simulink model "HLSDem_SetPoint"  (R2016b)
settings: configuration reference "CodeGenConfigSet" (kept outside this file)
values from neighbouring files (symbols this model uses):
  EPM_N_MAX = fi(10000,EngSpeed_rpm)    [init_HLSDem_SetPoint.m]    (also in init_HLSDem_SetPoint_SIL.m)
  HLSDem_dnSetPLoLimHiTrm_C = Calibration.Parameter    [init_HLSDem_SetPoint.m]    (also in init_HLSDem_SetPoint_SIL.m = Simulink.Parameter)
  HLSDem_dnSetPLoLimLoTrm_C = Calibration.Parameter    [init_HLSDem_SetPoint.m]    (also in init_HLSDem_SetPoint_SIL.m = Simulink.Parameter)
  HLSDem_facFdbkCANKick_C = Calibration.Parameter    [init_HLSDem_SetPoint.m]    (also in init_HLSDem_SetPoint_SIL.m = Simulink.Parameter)
  HLSDem_facFdbkDrvKick_C = Calibration.Parameter    [init_HLSDem_SetPoint.m]    (also in init_HLSDem_SetPoint_SIL.m = Simulink.Parameter)
  HLSDem_facFdbkHGG_C = Calibration.Parameter    [init_HLSDem_SetPoint.m]    (also in init_HLSDem_SetPoint_SIL.m = Simulink.Parameter)
  HLSDem_facFdbkLGG_C = Calibration.Parameter    [init_HLSDem_SetPoint.m]    (also in init_HLSDem_SetPoint_SIL.m = Simulink.Parameter)
  HLSDem_facFdbkMaxAcs_C = Calibration.Parameter    [init_HLSDem_SetPoint.m]    (also in init_HLSDem_SetPoint_SIL.m = Simulink.Parameter)
  HLSDem_facFdbkMaxSysErr_C = Calibration.Parameter    [init_HLSDem_SetPoint.m]    (also in init_HLSDem_SetPoint_SIL.m = Simulink.Parameter)
  HLSDem_facFdbkMaxTra_C = Calibration.Parameter    [init_HLSDem_SetPoint.m]    (also in init_HLSDem_SetPoint_SIL.m = Simulink.Parameter)
  HLSDem_facFdbkRed1_C = Calibration.Parameter    [init_HLSDem_SetPoint.m]    (also in init_HLSDem_SetPoint_SIL.m = Simulink.Parameter)
  HLSDem_facFdbkRed2_C = Calibration.Parameter    [init_HLSDem_SetPoint.m]    (also in init_HLSDem_SetPoint_SIL.m = Simulink.Parameter)
  HLSDem_facFdbkRed3_C = Calibration.Parameter    [init_HLSDem_SetPoint.m]    (also in init_HLSDem_SetPoint_SIL.m = Simulink.Parameter)
  HLSDem_facFdbkStrt_C = Calibration.Parameter    [init_HLSDem_SetPoint.m]    (also in init_HLSDem_SetPoint_SIL.m = Simulink.Parameter)
  HLSDem_facFdbkSysDgrt1_C = Calibration.Parameter    [init_HLSDem_SetPoint.m]    (also in init_HLSDem_SetPoint_SIL.m = Simulink.Parameter)
  HLSDem_facFdbkSysDgrt2_C = Calibration.Parameter    [init_HLSDem_SetPoint.m]    (also in init_HLSDem_SetPoint_SIL.m = Simulink.Parameter)
  HLSDem_facFdbkSysDgrt3_C = Calibration.Parameter    [init_HLSDem_SetPoint.m]    (also in init_HLSDem_SetPoint_SIL.m = Simulink.Parameter)
  HLSDem_facSetPLoFlt_C = Calibration.Parameter    [init_HLSDem_SetPoint.m]    (also in init_HLSDem_SetPoint_SIL.m = Simulink.Parameter)
  HLSDem_facTrqHiPT1_C = Calibration.Parameter    [init_HLSDem_SetPoint.m]    (also in init_HLSDem_SetPoint_SIL.m = Simulink.Parameter)
  HLSDem_facTrqLoPT1_C = Calibration.Parameter    [init_HLSDem_SetPoint.m]    (also in init_HLSDem_SetPoint_SIL.m = Simulink.Parameter)
  HLSDem_nHGGSetPHi_C = Calibration.Parameter    [init_HLSDem_SetPoint.m]    (also in init_HLSDem_SetPoint_SIL.m = Simulink.Parameter)
  HLSDem_nKDSetPHi_C = Calibration.Parameter    [init_HLSDem_SetPoint.m]    (also in init_HLSDem_SetPoint_SIL.m = Simulink.Parameter)
  HLSDem_nLGGSetPHi_C = Calibration.Parameter    [init_HLSDem_SetPoint.m]    (also in init_HLSDem_SetPoint_SIL.m = Simulink.Parameter)
  HLSDem_nRed1SetPHi_C = Calibration.Parameter    [init_HLSDem_SetPoint.m]    (also in init_HLSDem_SetPoint_SIL.m = Simulink.Parameter)
  HLSDem_nRed2SetPHi_C = Calibration.Parameter    [init_HLSDem_SetPoint.m]    (also in init_HLSDem_SetPoint_SIL.m = Simulink.Parameter)
  HLSDem_nRed3SetPHi_C = Calibration.Parameter    [init_HLSDem_SetPoint.m]    (also in init_HLSDem_SetPoint_SIL.m = Simulink.Parameter)
  HLSDem_nSel1SetPLo_C = Calibration.Parameter    [init_HLSDem_SetPoint.m]    (also in init_HLSDem_SetPoint_SIL.m = Simulink.Parameter)
  HLSDem_nSel2SetPLo_C = Calibration.Parameter    [init_HLSDem_SetPoint.m]    (also in init_HLSDem_SetPoint_SIL.m = Simulink.Parameter)
  HLSDem_nSel3SetPLo_C = Calibration.Parameter    [init_HLSDem_SetPoint.m]    (also in init_HLSDem_SetPoint_SIL.m = Simulink.Parameter)
  HLSDem_nSetPLoDia_C = Calibration.Parameter    [init_HLSDem_SetPoint.m]    (also in init_HLSDem_SetPoint_SIL.m = Simulink.Parameter)
  HLSDem_nSetPLoDrvAwy_C = Calibration.Parameter    [init_HLSDem_SetPoint.m]    (also in init_HLSDem_SetPoint_SIL.m = Simulink.Parameter)
  HLSDem_nSetPLoIni_CUR = Calibration.Parameter    [init_HLSDem_SetPoint.m]    (also in init_HLSDem_SetPoint_SIL.m = Simulink.Parameter)
  HLSDem_nSetPLoIni_CURX = Calibration.Parameter    [init_HLSDem_SetPoint.m]    (also in init_HLSDem_SetPoint_SIL.m = Simulink.Parameter)
  HLSDem_nSetPLoMax_C = Calibration.Parameter    [init_HLSDem_SetPoint.m]    (also in init_HLSDem_SetPoint_SIL.m = Simulink.Parameter)
  HLSDem_nSetPLoMaxOfs_C = Calibration.Parameter    [init_HLSDem_SetPoint.m]    (also in init_HLSDem_SetPoint_SIL.m = Simulink.Parameter)
  HLSDem_nSetPLoOfsMoF_C = Calibration.Parameter    [init_HLSDem_SetPoint.m]    (also in init_HLSDem_SetPoint_SIL.m = Simulink.Parameter)
  HLSDem_nSetPLoWrm_C = Calibration.Parameter    [init_HLSDem_SetPoint.m]    (also in init_HLSDem_SetPoint_SIL.m = Simulink.Parameter)
  HLSDem_nSpdLowBattUAdd_CUR = Calibration.Parameter    [init_HLSDem_SetPoint.m]    (also in init_HLSDem_SetPoint_SIL.m = Simulink.Parameter)
  HLSDem_nSpdLowBattUAdd_CURX = Calibration.Parameter    [init_HLSDem_SetPoint.m]    (also in init_HLSDem_SetPoint_SIL.m = Simulink.Parameter)
  HLSDem_nSpdLowBattUAddLim_C = Calibration.Parameter    [init_HLSDem_SetPoint.m]    (also in init_HLSDem_SetPoint_SIL.m = Simulink.Parameter)
  HLSDem_nStrtSetPHi_C = Calibration.Parameter    [init_HLSDem_SetPoint.m]    (also in init_HLSDem_SetPoint_SIL.m = Simulink.Parameter)
  HLSDem_nSysDgrtSetPHi_C = Calibration.Parameter    [init_HLSDem_SetPoint.m]    (also in init_HLSDem_SetPoint_SIL.m = Simulink.Parameter)
  HLSDem_rTrqSwt_C = Calibration.Parameter    [init_HLSDem_SetPoint.m]    (also in init_HLSDem_SetPoint_SIL.m = Simulink.Parameter)
  HLSDem_SetPHiRmpSlopeNeg_C = Calibration.Parameter    [init_HLSDem_SetPoint.m]    (also in init_HLSDem_SetPoint_SIL.m = Simulink.Parameter)
  HLSDem_SetPHiRmpSlopePos_C = Calibration.Parameter    [init_HLSDem_SetPoint.m]    (also in init_HLSDem_SetPoint_SIL.m = Simulink.Parameter)
  HLSDem_SetPLoRmpSlopeNeg_C = Calibration.Parameter    [init_HLSDem_SetPoint.m]    (also in init_HLSDem_SetPoint_SIL.m = Simulink.Parameter)
  HLSDem_SetPLoRmpSlopePos_C = Calibration.Parameter    [init_HLSDem_SetPoint.m]    (also in init_HLSDem_SetPoint_SIL.m = Simulink.Parameter)
  HLSDem_SetPLoTipInRmpSlopeNeg_C = Calibration.Parameter    [init_HLSDem_SetPoint.m]    (also in init_HLSDem_SetPoint_SIL.m = Simulink.Parameter)
  HLSDem_SetPLoTipInRmpSlopePos_C = Calibration.Parameter    [init_HLSDem_SetPoint.m]    (also in init_HLSDem_SetPoint_SIL.m = Simulink.Parameter)
  HLSDem_stSetPLoFlt_C = Calibration.Parameter    [init_HLSDem_SetPoint.m]    (also in init_HLSDem_SetPoint_SIL.m = Simulink.Parameter)
  HLSDem_stSpdSel_C = Calibration.Parameter    [init_HLSDem_SetPoint.m]    (also in init_HLSDem_SetPoint_SIL.m = Simulink.Parameter)
  HLSDem_stSysDgrtSetPHi_C = Calibration.Parameter    [init_HLSDem_SetPoint.m]    (also in init_HLSDem_SetPoint_SIL.m = Simulink.Parameter)
  HLSDem_swtDisblVehIfcSetPHi_C = Calibration.Parameter    [init_HLSDem_SetPoint.m]    (also in init_HLSDem_SetPoint_SIL.m = Simulink.Parameter)
  HLSDem_swtEnaPTO_C = Calibration.Parameter    [init_HLSDem_SetPoint.m]    (also in init_HLSDem_SetPoint_SIL.m = Simulink.Parameter)
  HLSDem_swtMode_C = Calibration.Parameter    [init_HLSDem_SetPoint.m]    (also in init_HLSDem_SetPoint_SIL.m = Simulink.Parameter)
  HLSDem_swtTempSel_C = Calibration.Parameter    [init_HLSDem_SetPoint.m]    (also in init_HLSDem_SetPoint_SIL.m = Simulink.Parameter)
  HLSDem_swtTrqHiSel_C = Calibration.Parameter    [init_HLSDem_SetPoint.m]    (also in init_HLSDem_SetPoint_SIL.m = Simulink.Parameter)
  HLSDem_swtTrqLoSel_C = Calibration.Parameter    [init_HLSDem_SetPoint.m]    (also in init_HLSDem_SetPoint_SIL.m = Simulink.Parameter)
  HLSDem_tDflSetPLo_C = Calibration.Parameter    [init_HLSDem_SetPoint.m]    (also in init_HLSDem_SetPoint_SIL.m = Simulink.Parameter)
  HLSDem_tiMaxIncrSetPLo_C = Calibration.Parameter    [init_HLSDem_SetPoint.m]    (also in init_HLSDem_SetPoint_SIL.m = Simulink.Parameter)
  HLSDem_tiSpdLowBattUAdd_C = Calibration.Parameter    [init_HLSDem_SetPoint.m]    (also in init_HLSDem_SetPoint_SIL.m = Simulink.Parameter)
  HLSDem_tiStrtCEngDsT_CUR = Calibration.Parameter    [init_HLSDem_SetPoint.m]    (also in init_HLSDem_SetPoint_SIL.m = Simulink.Parameter)
  HLSDem_tiStrtCEngDsT_CURX = Calibration.Parameter    [init_HLSDem_SetPoint.m]    (also in init_HLSDem_SetPoint_SIL.m = Simulink.Parameter)
  HLSDem_tiStrtEngOil_CUR = Calibration.Parameter    [init_HLSDem_SetPoint.m]    (also in init_HLSDem_SetPoint_SIL.m = Simulink.Parameter)
  HLSDem_tiStrtEngOil_CURX = Calibration.Parameter    [init_HLSDem_SetPoint.m]    (also in init_HLSDem_SetPoint_SIL.m = Simulink.Parameter)
  HLSDem_tThresDisbl_C = Calibration.Parameter    [init_HLSDem_SetPoint.m]    (also in init_HLSDem_SetPoint_SIL.m = Simulink.Parameter)
  HLSDem_tThresEna_C = Calibration.Parameter    [init_HLSDem_SetPoint.m]    (also in init_HLSDem_SetPoint_SIL.m = Simulink.Parameter)
  HLSDem_volSpdAddHi_C = Calibration.Parameter    [init_HLSDem_SetPoint.m]    (also in init_HLSDem_SetPoint_SIL.m = Simulink.Parameter)
  HLSDem_volSpdAddLo_C = Calibration.Parameter    [init_HLSDem_SetPoint.m]    (also in init_HLSDem_SetPoint_SIL.m = Simulink.Parameter)
  HndBrk_stDebVal_C = Calibration.Parameter    [init_HLSDem_SetPoint.m]    (also in init_HLSDem_SetPoint_SIL.m = Simulink.Parameter)
  SigTst_nSetPHi_C = Calibration.Parameter    [init_HLSDem_SetPoint.m]    (also in init_HLSDem_SetPoint_SIL.m = Simulink.Parameter)
  SigTst_nSetPLo_C = Calibration.Parameter    [init_HLSDem_SetPoint.m]    (also in init_HLSDem_SetPoint_SIL.m = Simulink.Parameter)
  SigTst_swtSetPHi_C = Calibration.Parameter    [init_HLSDem_SetPoint.m]    (also in init_HLSDem_SetPoint_SIL.m = Simulink.Parameter)
  SigTst_swtSetPLo_C = Calibration.Parameter    [init_HLSDem_SetPoint.m]    (also in init_HLSDem_SetPoint_SIL.m = Simulink.Parameter)
undefined symbols (not defined in the file or in its folder): CEngDst_switch_conv, CEngDsT_tTransf_CURX, EngState_conv, HLSDem_SetPoint_DT, StSys_StrtState_conv, Switch_conv
libraries: CXLib x13, simulink x3
(part 1 of 2)
settings Model: SimulationMode=accelerator  Creator=Administrator  LastModifiedBy=xuxingpei
settings ConfigSetRef: SourceLocation=Base Workspace

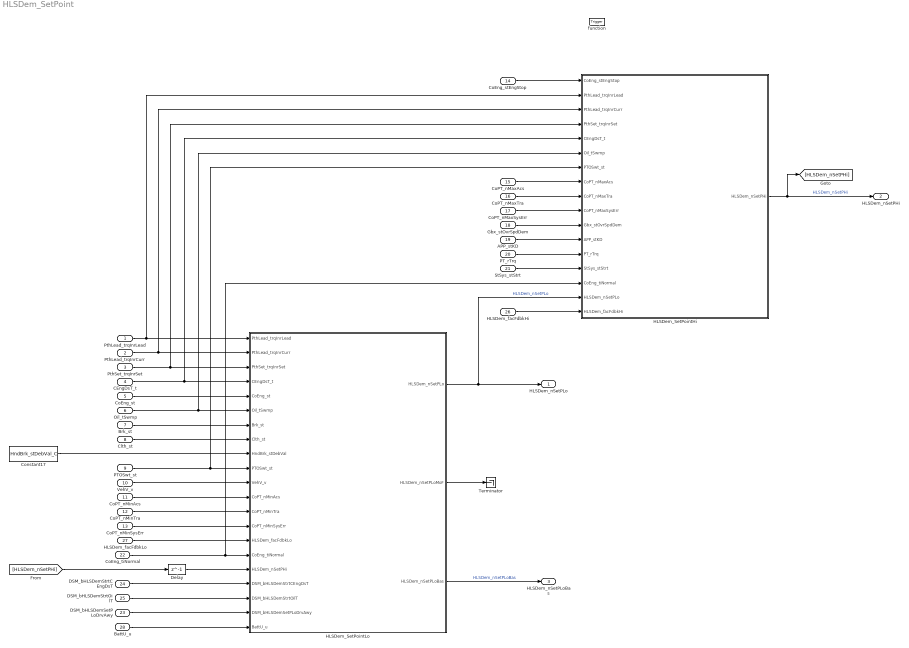
== system HLSDem_SetPoint ==
  PthLead_trqInrLead : Inport  Tag=Nm  Description=Inner torque lead value  OutMin=-3000  OutMax=3000  OutDataTypeStr=Trq_Nm
  PthLead_trqInrCurr : Inport  Tag=Nm  Description=Actual percent engine torque  Port=2  OutMin=-3000  OutMax=3000  OutDataTypeStr=Trq_Nm
  PthSet_trqInrSet : Inport  Tag=Nm  Description=Inner torque set value after monitoring limitation  Port=3  OutMin=-3000  OutMax=3276.7  OutDataTypeStr=Trq_Nm
  CEngDsT_t : Inport  Tag=deg  Description=engine coolant temperature after filter  Port=4  OutMin=-200  OutMax=200  OutDataTypeStr=Temp_deg
  CoEng_st : Inport  Description=Engine coordinator state  Port=5  OutDataTypeStr=Enum: EngState_conv
  Oil_tSwmp : Inport  Tag=deg  Description=Oil temperature in oil sump  Port=6  OutMin=-50  OutMax=200  OutDataTypeStr=Temp_deg
  Brk_st : Inport  Description=Brake switch state  Port=7  OutMin=0  OutMax=255  OutDataTypeStr=State_uint8
  Clth_st : Inport  Description=Clutch information  Port=8  OutMin=0  OutMax=255  OutDataTypeStr=State_uint8
  PTOSwt_st : Inport  Description=Power Take-off switch current state for a specific input voltage  Port=9  OutMin=0  OutMax=255  OutDataTypeStr=State_uint8
  VehV_v : Inport  Tag=km/h  Description=Vehicle speed  Port=10  OutMin=0  OutMax=250  OutDataTypeStr=VehSpeed_km_h
  CoPT_nMinAcs : Inport  Tag=rpm  Description=Application parameter for Minimum engine speed demand of Accessories  Port=11  OutMin=0  OutMax=6000  OutDataTypeStr=EngSpeed_rpm
  CoPT_nMinTra : Inport  Tag=rpm  Description=Application parameter for Minimum engine speed demand of transmission  Port=12  OutMin=0  OutMax=6000  OutDataTypeStr=EngSpeed_rpm
  CoPT_nMinSysErr : Inport  Tag=rpm  Description=Application parameter for Minimum engine speed demand while system error  Port=13  OutMin=0  OutMax=6000  OutDataTypeStr=EngSpeed_rpm
  CoEng_stEngStop : Inport  Description=Bit coded output message from engine stop function for low idle, egine shut off and crank control  Port=14  OutMin=0  OutMax=255  OutDataTypeStr=State_uint8
  CoPT_nMaxAcs : Inport  Tag=rpm  Description=Application parameter for maximum engine speed  Port=15  OutMin=0  OutMax=6000  OutDataTypeStr=EngSpeed_rpm
  CoPT_nMaxTra : Inport  Tag=rpm  Description=Application parameter for maximum engine speed demand of transmission  Port=16  OutMin=0  OutMax=6000  OutDataTypeStr=EngSpeed_rpm
  CoPT_nMaxSysErr : Inport  Tag=rpm  Description=Application parameter for maximum engine speed demand while system error  Port=17  OutMin=0  OutMax=6000  OutDataTypeStr=EngSpeed_rpm
  Gbx_stOvrSpdDem : Inport  Description=status of engine overspeed request  Port=18  OutMin=0  OutMax=255  OutDataTypeStr=State_uint8
  APP_stKD : Inport  Description=State of accelerator pedal kick down  Port=19  OutMin=0  OutMax=1  OutDataTypeStr=boolean
  PT_rTrq : Inport  Description=Powertrain torque ratio  Port=20  OutMin=-100  OutMax=100  OutDataTypeStr=TransRatio
  StSys_stStrt : Inport  Description=state of starting system  Port=21  OutDataTypeStr=Enum: StSys_StrtState_conv
  CoEng_tiNormal : Inport  Tag=ms  Description="Time since state\"CONENG_RUNNING\"was reached"  Port=22  OutMin=0  OutMax=42949672950  OutDataTypeStr=EngTime_ms
  DSM_bHLSDemSetPLoDrvAwy : Inport  Description=Status of FId_HLSDemSetPLoDrvAwy  Port=23  OutMin=0  OutMax=1  OutDataTypeStr=boolean
  DSM_bHLSDemStrtCEngDsT : Inport  Description=Status of FId_HLSDemStrtCEngDsT  Port=24  OutMin=0  OutMax=1  OutDataTypeStr=boolean
  DSM_bHLSDemStrtOilT : Inport  Description=Status of FId_HLSDemStrtOilT  Port=25  OutMin=0  OutMax=1  OutDataTypeStr=boolean
  HLSDem_facFdbkHi : Inport  Tag=rpm/Nm  Description=Feedback factor for the upper setpoint  Port=26  OutMin=-20  OutMax=20  OutDataTypeStr=FdbkNm2rpm_rpm_Nm
  HLSDem_facFdbkLo : Inport  Tag=rpm/Nm  Description=Feedback factor for the lower setpoint  Port=27  OutMin=-20  OutMax=20  OutDataTypeStr=FdbkNm2rpm_rpm_Nm
  BattU_u : Inport  Tag=mv  Description=Battery voltage  Port=28  OutMin=0  OutMax=50000  OutDataTypeStr=Battery_mv
  function : TriggerPort  TriggerType=function-call  VariantControl=Variant
  Constant17 : Constant  Value=HndBrk_stDebVal_C
  Delay : Delay  DelayLength=1  InitialCondition=0
  HLSDem_SetPointHi : Subsystem  RTWFcnName=HLSDem_SetPointHi_Co  RTWFileName=HLSDem
      settings: RTWSystemCode=Nonreusable function  RTWFcnNameOpts=User specified  RTWFileNameOpts=User specified
  HLSDem_SetPointLo : Subsystem  RequirementInfo="{}  %GIDa_cfd4d359_e493_4432_87ee_c1e2d06c7ea0"  RTWFcnName=HLSDem_SetPointLo_Co  RTWFileName=HLSDem
      settings: RTWSystemCode=Nonreusable function  RTWFcnNameOpts=User specified  RTWFileNameOpts=User specified
  Terminator : Terminator
  HLSDem_nSetPLo : Outport  Tag=rpm  Description=Minimum engine speed of HLSDem  OutMin=0  OutMax=6000  OutDataTypeStr=EngSpeed_rpm
  HLSDem_nSetPHi : Outport  Tag=rpm  Description=Maximum engine speed of HLSDem  Port=2  OutMin=0  OutMax=6000  OutDataTypeStr=EngSpeed_rpm
  HLSDem_nSetPLoBas : Outport  Tag=rpm  Description=Basic low idle setpoint speed (rpm)  Port=3  OutMin=0  OutMax=6000  OutDataTypeStr=EngSpeed_rpm
  wires:
  CEngDsT_t/1 -> HLSDem_SetPointLo/4(CEngDsT_t), HLSDem_SetPointHi/5(CEngDsT_t)
  CoEng_st/1 -> HLSDem_SetPointLo/5(CoEng_st)
  Oil_tSwmp/1 -> HLSDem_SetPointLo/6(Oil_tSwmp), HLSDem_SetPointHi/6(Oil_tSwmp)
  Brk_st/1 -> HLSDem_SetPointLo/7(Brk_st)
  Clth_st/1 -> HLSDem_SetPointLo/8(Clth_st)
  Constant17/1 -> HLSDem_SetPointLo/9(HndBrk_stDebVal)
  PTOSwt_st/1 -> HLSDem_SetPointLo/10(PTOSwt_st), HLSDem_SetPointHi/7(PTOSwt_st)
  HLSDem_SetPointHi/1(HLSDem_nSetPHi) -> HLSDem_nSetPHi/1, [HLSDem_nSetPHi]  "HLSDem_nSetPHi"
  PthLead_trqInrLead/1 -> HLSDem_SetPointLo/1(PthLead_trqInrLead), HLSDem_SetPointHi/2(PthLead_trqInrLead)
  PthLead_trqInrCurr/1 -> HLSDem_SetPointLo/2(PthLead_trqInrCurr), HLSDem_SetPointHi/3(PthLead_trqInrCurr)
  PthSet_trqInrSet/1 -> HLSDem_SetPointLo/3(PthSet_trqInrSet), HLSDem_SetPointHi/4(PthSet_trqInrSet)
  CoEng_stEngStop/1 -> HLSDem_SetPointHi/1(CoEng_stEngStop)
  StSys_stStrt/1 -> HLSDem_SetPointHi/14(StSys_stStrt)
  PT_rTrq/1 -> HLSDem_SetPointHi/13(PT_rTrq)
  APP_stKD/1 -> HLSDem_SetPointHi/12(APP_stKD)
  Gbx_stOvrSpdDem/1 -> HLSDem_SetPointHi/11(Gbx_stOvrSpdDem)
  CoPT_nMaxSysErr/1 -> HLSDem_SetPointHi/10(CoPT_nMaxSysErr)
  CoPT_nMaxTra/1 -> HLSDem_SetPointHi/9(CoPT_nMaxTra)
  CoPT_nMaxAcs/1 -> HLSDem_SetPointHi/8(CoPT_nMaxAcs)
  CoEng_tiNormal/1 -> HLSDem_SetPointLo/16(CoEng_tiNormal), HLSDem_SetPointHi/15(CoEng_tiNormal)
  HLSDem_SetPointLo/1(HLSDem_nSetPLo) -> HLSDem_SetPointHi/16(HLSDem_nSetPLo), HLSDem_nSetPLo/1  "HLSDem_nSetPLo"
  HLSDem_facFdbkHi/1 -> HLSDem_SetPointHi/17(HLSDem_facFdbkHi)
  HLSDem_SetPointLo/2(HLSDem_nSetPLoMoF) -> Terminator/1
  VehV_v/1 -> HLSDem_SetPointLo/11(VehV_v)
  CoPT_nMinAcs/1 -> HLSDem_SetPointLo/12(CoPT_nMinAcs)
  CoPT_nMinTra/1 -> HLSDem_SetPointLo/13(CoPT_nMinTra)
  CoPT_nMinSysErr/1 -> HLSDem_SetPointLo/14(CoPT_nMinSysErr)
  HLSDem_facFdbkLo/1 -> HLSDem_SetPointLo/15(HLSDem_facFdbkLo)
  DSM_bHLSDemStrtCEngDsT/1 -> HLSDem_SetPointLo/18(DSM_bHLSDemStrtCEngDsT)
  DSM_bHLSDemStrtOilT/1 -> HLSDem_SetPointLo/19(DSM_bHLSDemStrtOilT)
  DSM_bHLSDemSetPLoDrvAwy/1 -> HLSDem_SetPointLo/20(DSM_bHLSDemSetPLoDrvAwy)
  Delay/1 -> HLSDem_SetPointLo/17(HLSDem_nSetPHi)
  [HLSDem_nSetPHi] -> Delay/1
  HLSDem_SetPointLo/3(HLSDem_nSetPLoBas) -> HLSDem_nSetPLoBas/1  "HLSDem_nSetPLoBas"
  BattU_u/1 -> HLSDem_SetPointLo/21(BattU_u)

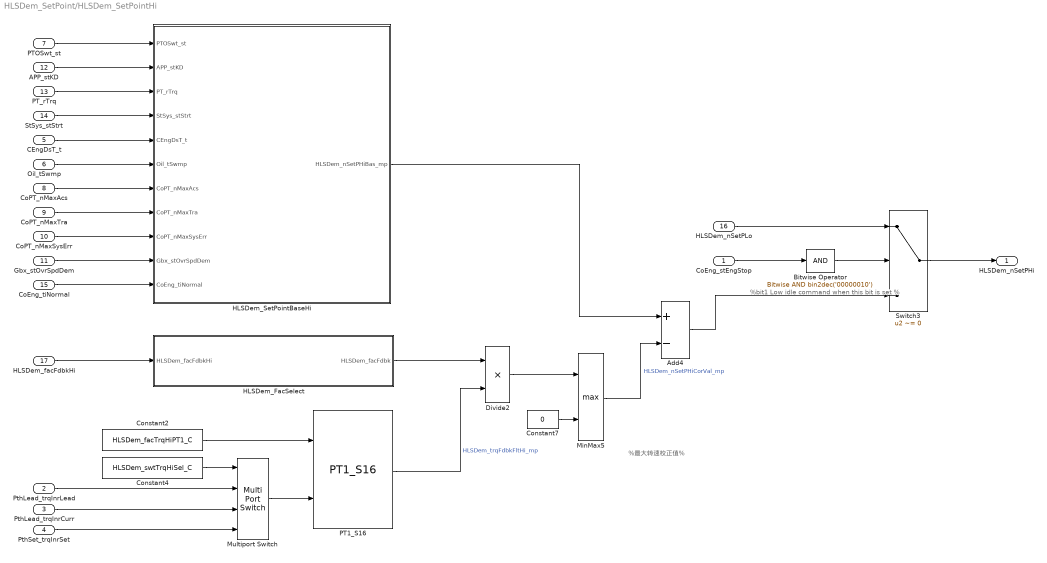
== system HLSDem_SetPoint/HLSDem_SetPointHi ==
  note: %bit1 Low idle command when this bit is set %
  note: %最大转速校正值%
  CoEng_stEngStop : Inport
  PthLead_trqInrLead : Inport  Port=2
  PthLead_trqInrCurr : Inport  Port=3
  PthSet_trqInrSet : Inport  Port=4
  CEngDsT_t : Inport  Port=5
  Oil_tSwmp : Inport  Port=6
  PTOSwt_st : Inport  Port=7
  CoPT_nMaxAcs : Inport  Port=8
  CoPT_nMaxTra : Inport  Port=9
  CoPT_nMaxSysErr : Inport  Port=10
  Gbx_stOvrSpdDem : Inport  Port=11
  APP_stKD : Inport  Port=12
  PT_rTrq : Inport  Port=13
  StSys_stStrt : Inport  Port=14
  CoEng_tiNormal : Inport  Port=15
  HLSDem_nSetPLo : Inport  Port=16
  HLSDem_facFdbkHi : Inport  Port=17
  Add4 : Sum  Inputs=+-  SaturateOnIntegerOverflow=on  InputSameDT=on
  Bitwise Operator : simulink/Logic and Bit Operations/Bitwise Operator  logicop=AND  UseBitMask=on  BitMask=bin2dec('00000010')  BitMaskRealWorld=Stored Integer
  Constant2 : Constant  Value=HLSDem_facTrqHiPT1_C
  Constant4 : Constant  Value=HLSDem_swtTrqHiSel_C
  Constant7 : Constant  Value=0  OutDataTypeStr=Inherit: Inherit via back propagation
  Divide2 : Product  Inputs=**  OutDataTypeStr=EngSpeed_rpm  SaturateOnIntegerOverflow=on
  HLSDem_FacSelect : Subsystem  RTWFcnName=HLSDem_FacSelect_Co  RTWFileName=HLSDem
      settings: RTWSystemCode=Nonreusable function  RTWFcnNameOpts=User specified  RTWFileNameOpts=User specified
  HLSDem_SetPointBaseHi : Subsystem  RTWFcnName=HLSDem_SetPointBaseHi_Co  RTWFileName=HLSDem_SetPointBaseHi
      settings: RTWSystemCode=Nonreusable function  RTWFcnNameOpts=User specified  RTWFileNameOpts=User specified
  MinMax5 : MinMax  Function=max  Inputs=2  SaturateOnIntegerOverflow=on  InputSameDT=on
  Multiport Switch : MultiPortSwitch  DataPortOrder=Specify indices  DataPortIndices={2,1,0}  SaturateOnIntegerOverflow=on  InputSameDT=on
  PT1_S16 : CXLib/PT1_S16  RequirementInfo={'other' 'HLSDem_SetPointHi_requirements.docx' '@Simulink_requirement_item_13' 'true' '扭矩滤波' '' } %GIDa_faa90fb1_26a3_42d9_b3d6_c3ce031b3aa7
  Switch3 : Switch  RequirementInfo={'other' 'HLSDem_SetPointHi_requirements.docx' '@Simulink_requirement_item_14' 'true' '目标最高转速选择' '' } %GIDa_8a0a6bc1_5cc4_4966_accb_2877bd54fcdc  Criteria=u2 ~= 0  SaturateOnIntegerOverflow=on  InputSameDT=on
  HLSDem_nSetPHi : Outport
  wires:
  HLSDem_facFdbkHi/1 -> HLSDem_FacSelect/1(HLSDem_facFdbkHi)
  CoEng_tiNormal/1 -> HLSDem_SetPointBaseHi/11(CoEng_tiNormal)
  Bitwise Operator/1 -> Switch3/2
  Multiport Switch/1 -> PT1_S16/2
  PT1_S16/1 -> Divide2/2  "HLSDem_trqFdbkFltHi_mp"
  Constant2/1 -> PT1_S16/1
  Switch3/1 -> HLSDem_nSetPHi/1
  CoEng_stEngStop/1 -> Bitwise Operator/1
  HLSDem_nSetPLo/1 -> Switch3/1
  Add4/1 -> Switch3/3
  MinMax5/1 -> Add4/2  "HLSDem_nSetPHiCorVal_mp"
  Divide2/1 -> MinMax5/1
  Constant7/1 -> MinMax5/2
  HLSDem_FacSelect/1(HLSDem_facFdbk) -> Divide2/1
  Constant4/1 -> Multiport Switch/1
  PthLead_trqInrLead/1 -> Multiport Switch/2
  PthLead_trqInrCurr/1 -> Multiport Switch/3
  PthSet_trqInrSet/1 -> Multiport Switch/4
  HLSDem_SetPointBaseHi/1(HLSDem_nSetPHiBas_mp) -> Add4/1
  Gbx_stOvrSpdDem/1 -> HLSDem_SetPointBaseHi/10(Gbx_stOvrSpdDem)
  CoPT_nMaxSysErr/1 -> HLSDem_SetPointBaseHi/9(CoPT_nMaxSysErr)
  CoPT_nMaxTra/1 -> HLSDem_SetPointBaseHi/8(CoPT_nMaxTra)
  CoPT_nMaxAcs/1 -> HLSDem_SetPointBaseHi/7(CoPT_nMaxAcs)
  PT_rTrq/1 -> HLSDem_SetPointBaseHi/3(PT_rTrq)
  PTOSwt_st/1 -> HLSDem_SetPointBaseHi/1(PTOSwt_st)
  APP_stKD/1 -> HLSDem_SetPointBaseHi/2(APP_stKD)
  StSys_stStrt/1 -> HLSDem_SetPointBaseHi/4(StSys_stStrt)
  CEngDsT_t/1 -> HLSDem_SetPointBaseHi/5(CEngDsT_t)
  Oil_tSwmp/1 -> HLSDem_SetPointBaseHi/6(Oil_tSwmp)

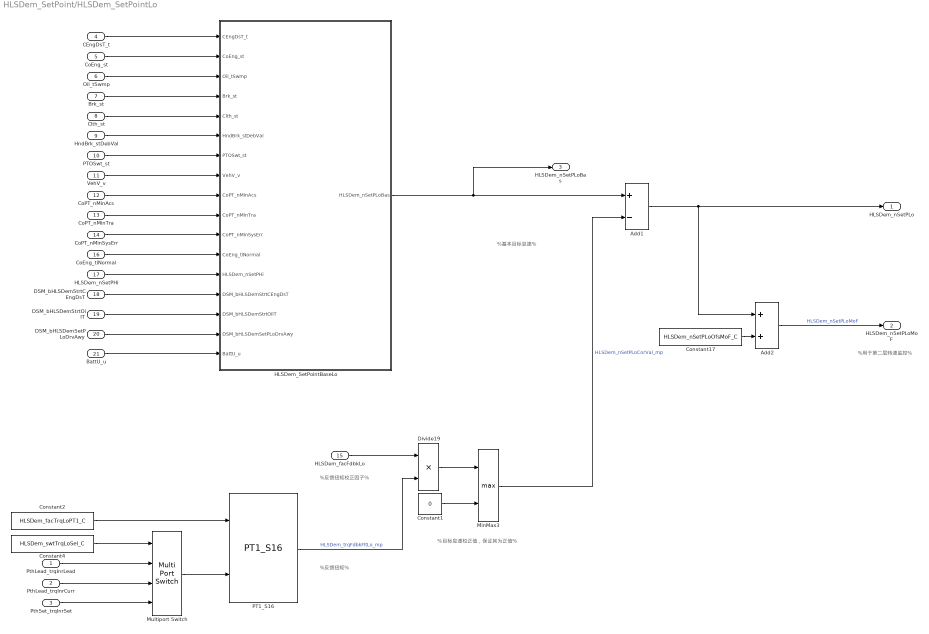
== system HLSDem_SetPoint/HLSDem_SetPointLo ==
  note: %基本目标怠速%
  note: %目标怠速校正值，保证其为正值%
  note: %反馈扭矩校正因子%
  note: %反馈扭矩%
  note: %用于第二层转速监控%
  PthLead_trqInrLead : Inport
  PthLead_trqInrCurr : Inport  Port=2
  PthSet_trqInrSet : Inport  Port=3
  CEngDsT_t : Inport  Port=4
  CoEng_st : Inport  Port=5
  Oil_tSwmp : Inport  Port=6
  Brk_st : Inport  Port=7
  Clth_st : Inport  Port=8
  HndBrk_stDebVal : Inport  Port=9
  PTOSwt_st : Inport  Port=10
  VehV_v : Inport  Port=11
  CoPT_nMinAcs : Inport  Port=12
  CoPT_nMinTra : Inport  Port=13
  CoPT_nMinSysErr : Inport  Port=14
  HLSDem_facFdbkLo : Inport  Port=15
  CoEng_tiNormal : Inport  Port=16
  HLSDem_nSetPHi : Inport  Port=17
  DSM_bHLSDemStrtCEngDsT : Inport  Port=18
  DSM_bHLSDemStrtOilT : Inport  Port=19
  DSM_bHLSDemSetPLoDrvAwy : Inport  Port=20
  BattU_u : Inport  Tag=mv  Description=Battery voltage  Port=21  OutMin=0  OutMax=50000  OutDataTypeStr=Battery_mv
  Add1 : Sum  Inputs=+-  SaturateOnIntegerOverflow=on  InputSameDT=on
  Add2 : Sum  RequirementInfo={'other' 'HLSDem_SetPointLo_requirements.docx' '@Simulink_requirement_item_13' 'true' '最终目标怠速及二级监控' '' } %GIDa_497d0e7b_cb5e_46b9_9089_a8d4edcec6b8  SaturateOnIntegerOverflow=on  InputSameDT=on
  Constant1 : Constant  Value=0  OutDataTypeStr=Inherit: Inherit via back propagation
  Constant17 : Constant  Value=HLSDem_nSetPLoOfsMoF_C
  Constant2 : Constant  Value=HLSDem_facTrqLoPT1_C
  Constant4 : Constant  Value=HLSDem_swtTrqLoSel_C
  Divide19 : Product  Inputs=**  OutDataTypeStr=EngSpeed_rpm  SaturateOnIntegerOverflow=on
  HLSDem_SetPointBaseLo : Subsystem  RequirementInfo={'other' 'HLSDem_SetPointLo_requirements.docx' '@Simulink_requirement_item_11' 'true' '目标怠速基础值计算' '' ; 'other' 'HLSDem_SetPointLo_requirements.docx' '@Simulink_requirement_item_11' 'true' '目标怠速基础值计算' '' } %GIDa_83b53250_afe4_4d04_87ea_d6290490e56f  RTWFcnName=HLSDem_SetPointBaseLo_Co  RTWFileName=HLSDem_SetPointBaseLo
      settings: RTWSystemCode=Nonreusable function  RTWFcnNameOpts=User specified  RTWFileNameOpts=User specified
  MinMax3 : MinMax  RequirementInfo={'other' 'HLSDem_SetPointLo_requirements.docx' '@Simulink_requirement_item_12' 'true' '目标怠速校正值计算' '' } %GIDa_59acb042_b405_4936_9c5b_c333c6a66b6e  Function=max  Inputs=2  SaturateOnIntegerOverflow=on  InputSameDT=on
  Multiport Switch : MultiPortSwitch  DataPortOrder=Specify indices  DataPortIndices={2,1,0}  SaturateOnIntegerOverflow=on  InputSameDT=on
  PT1_S16 : CXLib/PT1_S16
  HLSDem_nSetPLo : Outport
  HLSDem_nSetPLoMoF : Outport  Port=2
  HLSDem_nSetPLoBas : Outport  Port=3
  wires:
  CoEng_tiNormal/1 -> HLSDem_SetPointBaseLo/12(CoEng_tiNormal)
  PT1_S16/1 -> Divide19/2  "HLSDem_trqFdbkFltLo_mp"
  Constant2/1 -> PT1_S16/1
  Multiport Switch/1 -> PT1_S16/2
  PthLead_trqInrCurr/1 -> Multiport Switch/3
  MinMax3/1 -> Add1/2  "HLSDem_nSetPLoCorVal_mp"
  Constant4/1 -> Multiport Switch/1
  Add2/1 -> HLSDem_nSetPLoMoF/1  "HLSDem_nSetPLoMoF"
  PthLead_trqInrLead/1 -> Multiport Switch/2
  Divide19/1 -> MinMax3/1
  Constant1/1 -> MinMax3/2
  PthSet_trqInrSet/1 -> Multiport Switch/4
  Constant17/1 -> Add2/2
  CEngDsT_t/1 -> HLSDem_SetPointBaseLo/1(CEngDsT_t)
  CoEng_st/1 -> HLSDem_SetPointBaseLo/2(CoEng_st)
  HLSDem_facFdbkLo/1 -> Divide19/1
  HLSDem_nSetPHi/1 -> HLSDem_SetPointBaseLo/13(HLSDem_nSetPHi)
  VehV_v/1 -> HLSDem_SetPointBaseLo/8(VehV_v)
  PTOSwt_st/1 -> HLSDem_SetPointBaseLo/7(PTOSwt_st)
  HndBrk_stDebVal/1 -> HLSDem_SetPointBaseLo/6(HndBrk_stDebVal)
  Oil_tSwmp/1 -> HLSDem_SetPointBaseLo/3(Oil_tSwmp)
  HLSDem_SetPointBaseLo/1(HLSDem_nSetPLoBas) -> HLSDem_nSetPLoBas/1, Add1/1
  CoPT_nMinAcs/1 -> HLSDem_SetPointBaseLo/9(CoPT_nMinAcs)
  Add1/1 -> Add2/1, HLSDem_nSetPLo/1
  Brk_st/1 -> HLSDem_SetPointBaseLo/4(Brk_st)
  CoPT_nMinSysErr/1 -> HLSDem_SetPointBaseLo/11(CoPT_nMinSysErr)
  Clth_st/1 -> HLSDem_SetPointBaseLo/5(Clth_st)
  CoPT_nMinTra/1 -> HLSDem_SetPointBaseLo/10(CoPT_nMinTra)
  DSM_bHLSDemStrtCEngDsT/1 -> HLSDem_SetPointBaseLo/14(DSM_bHLSDemStrtCEngDsT)
  DSM_bHLSDemStrtOilT/1 -> HLSDem_SetPointBaseLo/15(DSM_bHLSDemStrtOilT)
  DSM_bHLSDemSetPLoDrvAwy/1 -> HLSDem_SetPointBaseLo/16(DSM_bHLSDemSetPLoDrvAwy)
  BattU_u/1 -> HLSDem_SetPointBaseLo/17(BattU_u)

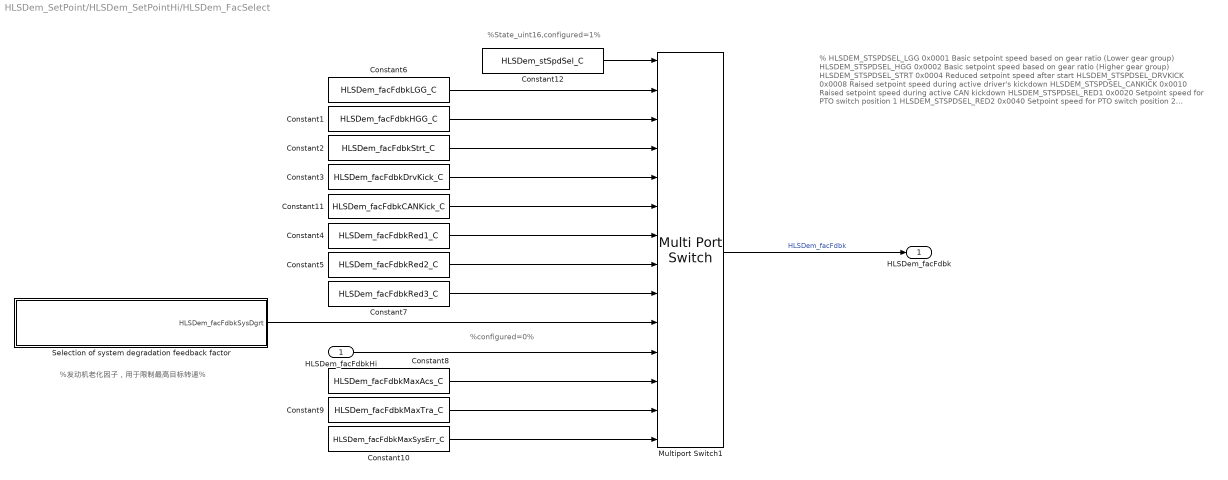
== system HLSDem_SetPoint/HLSDem_SetPointHi/HLSDem_FacSelect ==
  note: %发动机老化因子，用于限制最高目标转速%
  note: %
      | HLSDEM_STSPDSEL_LGG 0x0001 Basic setpoint speed based on gear ratio (Lower gear group)
      | HLSDEM_STSPDSEL_HGG 0x0002 Basic setpoint speed based on gear ratio (Higher gear group)
      | HLSDEM_STSPDSEL_STRT 0x0004 Reduced setpoint speed after start
      | HLSDEM_STSPDSEL_DRVKICK 0x0008 Raised setpoint speed during active driver's kickdown
      | HLSDEM_STSPDSEL_CANKICK 0x0010 Raised setpoint speed during active CAN kickdown
      | HLSDEM_STSPDSEL_RED1 0x0020 Setpoint speed for PTO switch position 1
      | HLSDEM_STSPDSEL_RED2 0x0040 Setpoint speed for PTO switch position 2
      | HLSDEM_STSPDSEL_RED3 0x0080 Setpoint speed for PTO switch position 3
      | HLSDEM_STSPDSEL_SYSDGRT 0x0100 Reduced setpoint speed from system degradation logic
      | HLSDEM_STSPDSEL_CAN 0x0200 Reduced setpoint speed via CAN (refer hlsdem_setpoint_var2_ml_fs.xml)
      | HLSDEM_STSPDSEL_ACS 0x0400 Setpoint speed of accessories (CoPT_nMaxAcs).
      | HLSDEM_STSPDSEL_TRA 0x0800 Setpoint speed of Transmission (CoPT_nMaxTra)
      | HLSDEM_STSPDSEL_SYSERR 0x1000 Setpoint speed during system error from vehicle (CoPT_nMaxSysErr) %
  note: %State_uint16,configured=1%
  note: %configured=0%
  HLSDem_facFdbkHi : Inport
  Constant1 : Constant  Value=HLSDem_facFdbkHGG_C
  Constant10 : Constant  Value=HLSDem_facFdbkMaxSysErr_C
  Constant11 : Constant  Value=HLSDem_facFdbkCANKick_C
  Constant12 : Constant  Value=HLSDem_stSpdSel_C
  Constant2 : Constant  Value=HLSDem_facFdbkStrt_C
  Constant3 : Constant  Value=HLSDem_facFdbkDrvKick_C
  Constant4 : Constant  Value=HLSDem_facFdbkRed1_C
  Constant5 : Constant  Value=HLSDem_facFdbkRed2_C
  Constant6 : Constant  Value=HLSDem_facFdbkLGG_C
  Constant7 : Constant  Value=HLSDem_facFdbkRed3_C
  Constant8 : Constant  Value=HLSDem_facFdbkMaxAcs_C
  Constant9 : Constant  Value=HLSDem_facFdbkMaxTra_C
  Multiport Switch1 : MultiPortSwitch  RequirementInfo={'other' 'HLSDem_FacSelect_requirements.docx' '@Simulink_requirement_item_2' 'true' '基于状态的调整系数选择' '' } %GIDa_1bc398cb_8e7c_43cb_a21c_2ea3ebed9f4a  DataPortOrder=Specify indices  Inputs=12  DataPortIndices={1,2,4,8,16,32,64,128,256,512,1024,2048,4096}  SaturateOnIntegerOverflow=on  InputSameDT=on
  Selection of system degradation feedback factor : Subsystem
  HLSDem_facFdbk : Outport
  wires:
  Constant11/1 -> Multiport Switch1/6
  Constant12/1 -> Multiport Switch1/1
  Multiport Switch1/1 -> HLSDem_facFdbk/1  "HLSDem_facFdbk"
  Constant6/1 -> Multiport Switch1/2
  Constant1/1 -> Multiport Switch1/3
  Constant2/1 -> Multiport Switch1/4
  Constant3/1 -> Multiport Switch1/5
  Constant4/1 -> Multiport Switch1/7
  Constant5/1 -> Multiport Switch1/8
  Constant7/1 -> Multiport Switch1/9
  HLSDem_facFdbkHi/1 -> Multiport Switch1/11
  Constant8/1 -> Multiport Switch1/12
  Constant9/1 -> Multiport Switch1/13
  Constant10/1 -> Multiport Switch1/14
  Selection of system degradation feedback factor/1(HLSDem_facFdbkSysDgrt) -> Multiport Switch1/10

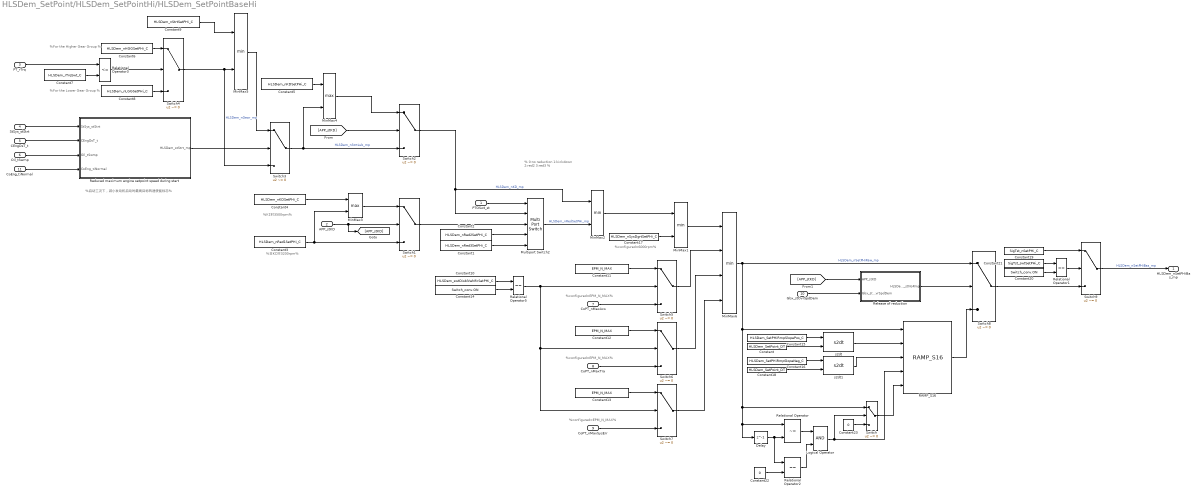
== system HLSDem_SetPoint/HLSDem_SetPointHi/HLSDem_SetPointBaseHi ==
  note: %configured=EPM_N_MAX%
  note: %configured=EPM_N_MAX%
  note: %
      | 0:no reduction
      | 1:kickdown
      | 2:red2
      | 3:red3
      | %
  note: %启动工况下，减小发动机启动时最高目标转速使能标志%
  note: %configured=EPM_N_MAX%
  note: %configured=6000rpm%
  note: %KD时3500rpm%
  note: %非KD时3200rpm%
  note: %For the Higher Gear Group %
  note: %For the Lower Gear Group %
  PTOSwt_st : Inport
  APP_stKD : Inport  Port=2
  PT_rTrq : Inport  Port=3
  StSys_stStrt : Inport  Port=4
  CEngDsT_t : Inport  Port=5
  Oil_tSwmp : Inport  Port=6
  CoPT_nMaxAcs : Inport  Port=7
  CoPT_nMaxTra : Inport  Port=8
  CoPT_nMaxSysErr : Inport  Port=9
  Gbx_stOvrSpdDem : Inport  Port=10
  CoEng_tiNormal : Inport  Port=11
  Constant : Constant  Value=HLSDem_SetPoint_DT
  Constant1 : Constant  Value=HLSDem_nRed3SetPHi_C
  Constant10 : Constant  Value=HLSDem_swtDisblVehIfcSetPHi_C
  Constant11 : Constant  Value=EPM_N_MAX  OutDataTypeStr=Inherit: Inherit via back propagation
  Constant12 : Constant  Value=EPM_N_MAX  OutDataTypeStr=Inherit: Inherit via back propagation
  Constant13 : Constant  Value=EPM_N_MAX  OutDataTypeStr=Inherit: Inherit via back propagation
  Constant14 : Constant  RequirementInfo={'other' 'APP_requirements.doc' '@Simulink_requirement_item_25' 'true' '手动开关' '' } %GIDa_eb49d9c2_e05e_4ab9_a401_029124554a49  Value=Switch_conv.ON  OutDataTypeStr=Inherit: Inherit via back propagation
  Constant15 : Constant  Value=HLSDem_SetPHiRmpSlopePos_C
  Constant16 : Constant  Value=HLSDem_SetPHiRmpSlopeNeg_C
  Constant17 : Constant  Value=HLSDem_nSysDgrtSetPHi_C
  Constant18 : Constant  Value=HLSDem_SetPoint_DT
  Constant19 : Constant  RequirementInfo={'other' 'CEngDsT_requirements.doc' '@Simulink_requirement_item_6' 'true' '手动冷却水温值' '' } %GIDa_93d9a20b_cefd_4ed3_96f3_664cd11dd16f  Value=SigTst_nSetPHi_C  SampleTime=-1
  Constant2 : Constant  Value=HLSDem_nRed2SetPHi_C
  Constant20 : Constant  RequirementInfo={'other' 'APP_requirements.doc' '@Simulink_requirement_item_25' 'true' '手动开关' '' } %GIDa_61b3e37d_447d_4b6a_bc06_d36a4fd8bafd  Value=Switch_conv.ON  OutDataTypeStr=Inherit: Inherit via back propagation
  Constant21 : Constant  RequirementInfo={'other' 'CEngDsT_requirements.doc' '@Simulink_requirement_item_6' 'true' '手动冷却水温值' '' } %GIDa_92fd4f01_8b91_4b12_9d10_1e37be35c0be  Value=SigTst_swtSetPHi_C  SampleTime=-1
  Constant22 : Constant  Value=0  OutDataTypeStr=Inherit: Inherit via back propagation
  Constant23 : Constant  Value=0  OutDataTypeStr=Inherit: Inherit via back propagation
  Constant3 : Constant  Value=HLSDem_nRed1SetPHi_C
  Constant4 : Constant  Value=HLSDem_nKDSetPHi_C
  Constant5 : Constant  Value=HLSDem_nKDSetPHi_C
  Constant6 : Constant  Value=HLSDem_nHGGSetPHi_C
  Constant7 : Constant  Value=HLSDem_rTrqSwt_C
  Constant8 : Constant  Value=HLSDem_nLGGSetPHi_C
  Constant9 : Constant  Value=HLSDem_nStrtSetPHi_C
  Delay : Delay  DelayLength=1  InitialCondition=0
  Logical Operator : Logic  AllPortsSameDT=off  OutDataTypeStr=boolean
  MinMax1 : MinMax  Inputs=2  SaturateOnIntegerOverflow=on  InputSameDT=on
  MinMax2 : MinMax  Inputs=2  SaturateOnIntegerOverflow=on  InputSameDT=on
  MinMax3 : MinMax  Function=max  Inputs=2  SaturateOnIntegerOverflow=on  InputSameDT=on
  MinMax4 : MinMax  Function=max  Inputs=2  SaturateOnIntegerOverflow=on  InputSameDT=on
  MinMax5 : MinMax  Inputs=2  SaturateOnIntegerOverflow=on  InputSameDT=on
  MinMax6 : MinMax  Inputs=4  SaturateOnIntegerOverflow=on  InputSameDT=on
  Multiport Switch2 : MultiPortSwitch  DataPortOrder=Zero-based contiguous  Inputs=4  SaturateOnIntegerOverflow=on  InputSameDT=on
  RAMP_S16 : CXLib/RAMP_S16  RequirementInfo={'other' 'HLSDem_SetPointHi_requirements.docx' '@Simulink_requirement_item_15' 'true' '转速斜坡过渡' '' } %GIDa_4caeb529_2a7a_4d64_ad60_570c507ee356
  Reduced maximum engine setpoint speed during start : Subsystem
  Relational Operator : RelationalOperator  Operator=~=  OutDataTypeStr=boolean  RndMeth=Simplest
  Relational Operator1 : RelationalOperator  Operator===  OutDataTypeStr=boolean  RndMeth=Simplest  InputSameDT=on
  Relational Operator2 : RelationalOperator  Operator===  OutDataTypeStr=boolean  RndMeth=Simplest  InputSameDT=on
  Relational Operator3 : RelationalOperator  Operator=<=  OutDataTypeStr=boolean  RndMeth=Nearest  InputSameDT=on
  Relational Operator5 : RelationalOperator  Operator===  OutDataTypeStr=boolean  RndMeth=Simplest  InputSameDT=on
  Release of reduction : Subsystem
  Switch : Switch  Criteria=u2 ~= 0  InputSameDT=on
  Switch{1..7} (7 alike) : Switch  Criteria=u2 ~= 0  SaturateOnIntegerOverflow=on  InputSameDT=on
  Switch8 : Switch  RequirementInfo={'other' 'HLSDem_SetPointHi_requirements.docx' '@Simulink_requirement_item_16' 'true' '目标最高转速选择' '' } %GIDa_22306cf8_a5c4_44a2_806f_afaba1cae9ca  Criteria=u2 ~= 0  SaturateOnIntegerOverflow=on  InputSameDT=on
  Switch9 : Switch  RequirementInfo={'other' 'CEngDsT_requirements.doc' '@Simulink_requirement_item_6' 'true' '手动冷却水温值' '' } %GIDa_9b48b579_1aec_4024_86bf_b27f3ab8e09f  Criteria=u2 ~= 0  Threshold=CEngDst_switch_conv.OFF  SaturateOnIntegerOverflow=on  InputSameDT=on
  s2dt : CXLib/s2dt
  s2dt1 : CXLib/s2dt
  HLSDem_nSetPHiBas_mp : Outport
  wires:
  Switch8/1 -> Switch9/3
  Constant20/1 -> Relational Operator1/2
  Constant21/1 -> Relational Operator1/1
  Relational Operator1/1 -> Switch9/2
  Constant19/1 -> Switch9/1
  s2dt1/1 -> RAMP_S16/3
  s2dt/1 -> RAMP_S16/2
  Constant15/1 -> s2dt/1
  Constant16/1 -> s2dt1/1
  Constant/1 -> s2dt/2
  Constant18/1 -> s2dt1/2
  CoEng_tiNormal/1 -> Reduced maximum engine setpoint speed during start/4(CoEng_tiNormal)
  Constant14/1 -> Relational Operator5/2
  Constant10/1 -> Relational Operator5/1
  Relational Operator5/1 -> Switch6/2, Switch7/2, Switch5/2
  RAMP_S16/1 -> Switch8/3
  MinMax6/1 -> RAMP_S16/1, Switch/1, Relational Operator/1, Delay/1, Switch8/1  "HLSDem_nSetPHiRaw_mp"
  MinMax2/1 -> MinMax1/1
  Constant17/1 -> MinMax1/2
  Multiport Switch2/1 -> MinMax2/2  "HLSDem_nRedSetPHi_mp"
  PTOSwt_st/1 -> Multiport Switch2/1
  Constant1/1 -> Multiport Switch2/5
  Constant2/1 -> Multiport Switch2/4
  Switch1/1 -> Multiport Switch2/3
  APP_stKD/1 -> [APP_stKD], Switch1/2
  MinMax3/1 -> Switch1/1
  Constant3/1 -> MinMax3/2, Switch1/3
  Constant4/1 -> MinMax3/1
  [APP_stKD] -> Switch2/2
  MinMax4/1 -> Switch2/1
  Switch2/1 -> MinMax2/1, Multiport Switch2/2  "HLSDem_nKD_mp"
  Switch3/1 -> MinMax4/2, Switch2/3  "HLSDem_nStrtLub_mp"
  Constant5/1 -> MinMax4/1
  Reduced maximum engine setpoint speed during start/1(HLSDem_stStrt_mp) -> Switch3/2
  MinMax5/1 -> Switch3/1
  Switch4/1 -> MinMax5/2, Switch3/3  "HLSDem_nGear_mp"
  Relational Operator3/1 -> Switch4/2
  PT_rTrq/1 -> Relational Operator3/1
  Constant7/1 -> Relational Operator3/2
  Constant6/1 -> Switch4/1
  Constant8/1 -> Switch4/3
  Constant9/1 -> MinMax5/1
  CEngDsT_t/1 -> Reduced maximum engine setpoint speed during start/2(CEngDsT_t)
  StSys_stStrt/1 -> Reduced maximum engine setpoint speed during start/1(StSys_stStrt)
  Oil_tSwmp/1 -> Reduced maximum engine setpoint speed during start/3(Oil_tSwmp)
  MinMax1/1 -> MinMax6/1
  Constant11/1 -> Switch5/1
  CoPT_nMaxAcs/1 -> Switch5/3
  Constant12/1 -> Switch6/1
  CoPT_nMaxTra/1 -> Switch6/3
  Switch6/1 -> MinMax6/3
  Constant13/1 -> Switch7/1
  CoPT_nMaxSysErr/1 -> Switch7/3
  Switch7/1 -> MinMax6/4
  Release of reduction/1(HLSDem_stNoRmp) -> Switch8/2
  Switch9/1 -> HLSDem_nSetPHiBas_mp/1  "HLSDem_nSetPHiBas_mp"
  Gbx_stOvrSpdDem/1 -> Release of reduction/2(Gbx_stOvrSpdDem)
  [APP_stKD] -> Release of reduction/1(APP_stKD)
  Switch5/1 -> MinMax6/2
  Logical Operator/1 -> RAMP_S16/4, Switch/2
  Delay/1 -> Relational Operator2/1, Relational Operator/2
  Relational Operator/1 -> Logical Operator/1
  Relational Operator2/1 -> Logical Operator/2
  Constant22/1 -> Relational Operator2/2
  Constant23/1 -> Switch/3
  Switch/1 -> RAMP_S16/5

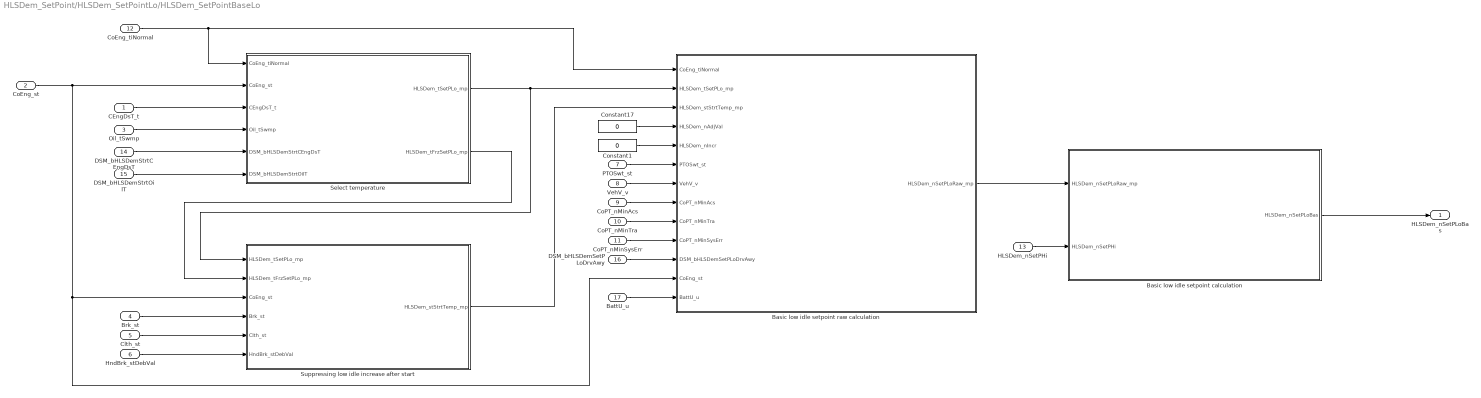
== system HLSDem_SetPoint/HLSDem_SetPointLo/HLSDem_SetPointBaseLo ==
  CEngDsT_t : Inport
  CoEng_st : Inport  Port=2
  Oil_tSwmp : Inport  Port=3
  Brk_st : Inport  Port=4
  Clth_st : Inport  Port=5
  HndBrk_stDebVal : Inport  Port=6
  PTOSwt_st : Inport  Port=7
  VehV_v : Inport  Port=8
  CoPT_nMinAcs : Inport  Port=9
  CoPT_nMinTra : Inport  Port=10
  CoPT_nMinSysErr : Inport  Port=11
  CoEng_tiNormal : Inport  Port=12
  HLSDem_nSetPHi : Inport  Port=13
  DSM_bHLSDemStrtCEngDsT : Inport  Port=14
  DSM_bHLSDemStrtOilT : Inport  Port=15
  DSM_bHLSDemSetPLoDrvAwy : Inport  Port=16
  BattU_u : Inport  Tag=mv  Description=Battery voltage  Port=17  OutMin=0  OutMax=50000  OutDataTypeStr=Battery_mv
  Basic low idle setpoint calculation : Subsystem  RequirementInfo={'other' 'HLSDem_SetPointLo_requirements.docx' '@Simulink_requirement_item_18' 'true' '目标怠速初始值计算' '' } %GIDa_48f1ce4a_a6d0_4006_a4e1_206a8b4b1f7d
  Basic low idle setpoint raw calculation : Subsystem
  Constant1 : Constant  Value=0  OutDataTypeStr=Inherit: Inherit via back propagation
  Constant17 : Constant  Value=0  OutDataTypeStr=Inherit: Inherit via back propagation
  Select temperature : Subsystem  RequirementInfo={'other' 'HLSDem_SetPointLo_requirements.docx' '@Simulink_requirement_item_14' 'true' '选择温度' '' } %GIDa_7b06c331_92b1_4ce7_a661_30450cc9a024
  Suppressing low idle increase after start : Subsystem  RequirementInfo={'other' 'HLSDem_SetPointLo_requirements.docx' '@Simulink_requirement_item_17' 'true' '抑制转速增加的限制性条件' '' } %GIDa_a792367d_af75_4b62_9cc7_000f1dba428d
  HLSDem_nSetPLoBas : Outport
  wires:
  CoEng_tiNormal/1 -> Select temperature/1(CoEng_tiNormal), Basic low idle setpoint raw calculation/1(CoEng_tiNormal)
  HLSDem_nSetPHi/1 -> Basic low idle setpoint calculation/2(HLSDem_nSetPHi)
  Constant17/1 -> Basic low idle setpoint raw calculation/4(HLSDem_nAdjVal)
  CoPT_nMinSysErr/1 -> Basic low idle setpoint raw calculation/10(CoPT_nMinSysErr)
  CoPT_nMinTra/1 -> Basic low idle setpoint raw calculation/9(CoPT_nMinTra)
  CoPT_nMinAcs/1 -> Basic low idle setpoint raw calculation/8(CoPT_nMinAcs)
  VehV_v/1 -> Basic low idle setpoint raw calculation/7(VehV_v)
  Constant1/1 -> Basic low idle setpoint raw calculation/5(HLSDem_nIncr)
  PTOSwt_st/1 -> Basic low idle setpoint raw calculation/6(PTOSwt_st)
  HndBrk_stDebVal/1 -> Suppressing low idle increase after start/6(HndBrk_stDebVal)
  Clth_st/1 -> Suppressing low idle increase after start/5(Clth_st)
  Brk_st/1 -> Suppressing low idle increase after start/4(Brk_st)
  Oil_tSwmp/1 -> Select temperature/4(Oil_tSwmp)
  CEngDsT_t/1 -> Select temperature/3(CEngDsT_t)
  Select temperature/2(HLSDem_tFrzSetPLo_mp) -> Suppressing low idle increase after start/2(HLSDem_tFrzSetPLo_mp)
  Basic low idle setpoint calculation/1(HLSDem_nSetPLoBas) -> HLSDem_nSetPLoBas/1
  Basic low idle setpoint raw calculation/1(HLSDem_nSetPLoRaw_mp) -> Basic low idle setpoint calculation/1(HLSDem_nSetPLoRaw_mp)
  Suppressing low idle increase after start/1(HLSDem_stStrtTemp_mp) -> Basic low idle setpoint raw calculation/3(HLSDem_stStrtTemp_mp)
  Select temperature/1(HLSDem_tSetPLo_mp) -> Basic low idle setpoint raw calculation/2(HLSDem_tSetPLo_mp), Suppressing low idle increase after start/1(HLSDem_tSetPLo_mp)
  DSM_bHLSDemStrtCEngDsT/1 -> Select temperature/5(DSM_bHLSDemStrtCEngDsT)
  DSM_bHLSDemStrtOilT/1 -> Select temperature/6(DSM_bHLSDemStrtOilT)
  DSM_bHLSDemSetPLoDrvAwy/1 -> Basic low idle setpoint raw calculation/11(DSM_bHLSDemSetPLoDrvAwy)
  BattU_u/1 -> Basic low idle setpoint raw calculation/13(BattU_u)
  CoEng_st/1 -> Select temperature/2(CoEng_st), Basic low idle setpoint raw calculation/12(CoEng_st), Suppressing low idle increase after start/3(CoEng_st)

== system HLSDem_SetPoint/HLSDem_SetPointHi/HLSDem_FacSelect/Selection of system degradation feedback factor ==
  note: %State_uint8,configured=defualt value (0)%
  Constant1 : Constant  Value=HLSDem_facFdbkSysDgrt2_C  SampleTime=-1
  Constant11 : Constant  Value=HLSDem_facFdbkSysDgrt3_C  SampleTime=-1
  Constant2 : Constant  Value=HLSDem_facFdbkSysDgrt1_C  SampleTime=-1
  Constant3 : Constant  Value=0  OutDataTypeStr=Inherit: Inherit via back propagation  SampleTime=-1
  Constant4 : Constant  Value=HLSDem_stSysDgrtSetPHi_C  SampleTime=-1
  Multiport Switch2 : MultiPortSwitch  RequirementInfo={'other' 'HLSDem_FacSelect_requirements.docx' '@Simulink_requirement_item_1' 'true' '基于系统老化的调整系数' '' } %GIDa_f470d177_122a_4567_8a2f_49a514bb53bd  DataPortOrder=Specify indices  Inputs=4  DataPortIndices={3,2,1,0}  InputSameDT=on
  HLSDem_facFdbkSysDgrt : Outport
  wires:
  Constant11/1 -> Multiport Switch2/2
  Constant1/1 -> Multiport Switch2/3
  Constant2/1 -> Multiport Switch2/4
  Constant3/1 -> Multiport Switch2/5
  Constant4/1 -> Multiport Switch2/1
  Multiport Switch2/1 -> HLSDem_facFdbkSysDgrt/1  "HLSDem_facFdbkSysDgrt"

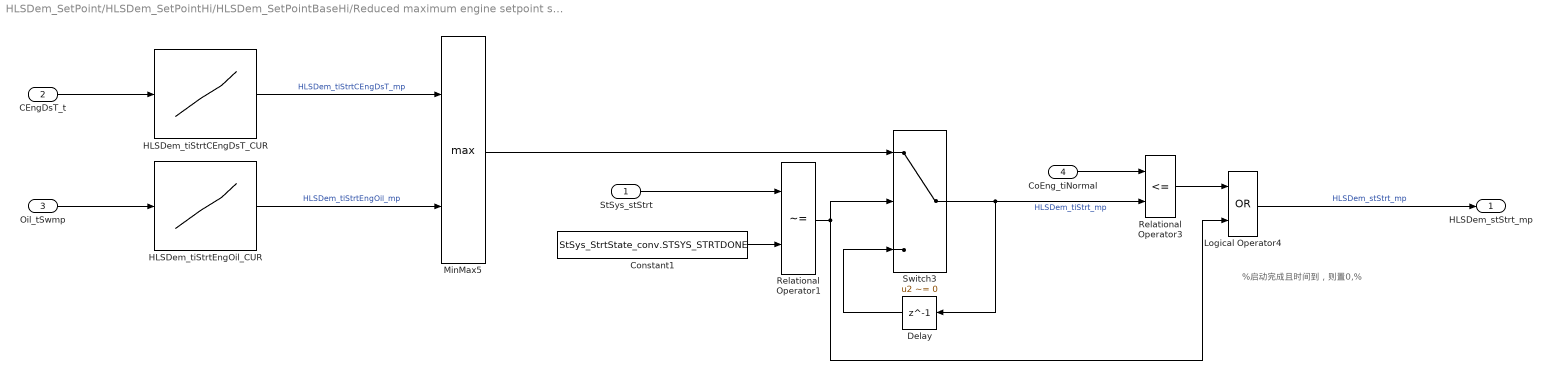
== system HLSDem_SetPoint/HLSDem_SetPointHi/HLSDem_SetPointBaseHi/Reduced maximum engine setpoint speed during start ==
  note: %启动完成且时间到，则置0,%
  StSys_stStrt : Inport
  CEngDsT_t : Inport  Port=2
  Oil_tSwmp : Inport  Port=3
  CoEng_tiNormal : Inport  Port=4
  Constant1 : Constant  Value=StSys_StrtState_conv.STSYS_STRTDONE
  Delay : Delay  DelayLength=1  InitialCondition=0
  HLSDem_tiStrtCEngDsT_CUR : Lookup_n-D  DialogController=Simulink.DDGSource  NumberOfTableDimensions=1  BreakpointsForDimension1=HLSDem_tiStrtCEngDsT_CURX  BreakpointsForDimension2=CEngDsT_tTransf_CURX  IndexSearchMethod=Linear search  BeginIndexSearchUsingPreviousIndexResult=on  Table=HLSDem_tiStrtCEngDsT_CUR  ExtrapMethod=Clip  UseLastTableValue=on  InternalRulePriority=Speed  OutDataTypeStr=Inherit: Inherit via back propagation  SaturateOnIntegerOverflow=on
  HLSDem_tiStrtEngOil_CUR : Lookup_n-D  DialogController=Simulink.DDGSource  NumberOfTableDimensions=1  BreakpointsForDimension1=HLSDem_tiStrtEngOil_CURX  BreakpointsForDimension2=CEngDsT_tTransf_CURX  IndexSearchMethod=Linear search  BeginIndexSearchUsingPreviousIndexResult=on  Table=HLSDem_tiStrtEngOil_CUR  ExtrapMethod=Clip  UseLastTableValue=on  InternalRulePriority=Speed  OutDataTypeStr=Inherit: Inherit via back propagation  SaturateOnIntegerOverflow=on
  Logical Operator4 : Logic  RequirementInfo={'other' 'HLSDem_SetPointHi_requirements.docx' '@Simulink_requirement_item_17' 'true' '启用启动状态最高设定转速状态判定' '' } %GIDa_1453ccb3_4a3d_46ad_8a77_b07e54f5156f  Operator=OR  OutDataTypeStr=boolean
  MinMax5 : MinMax  Function=max  Inputs=2  SaturateOnIntegerOverflow=on  InputSameDT=on
  Relational Operator1 : RelationalOperator  RequirementInfo={'other' 'HLSDem_SetPointHi_requirements.docx' '@Simulink_requirement_item_17' 'true' '启用启动状态最高设定转速状态判定' '' } %GIDa_45e5b883_16f9_45fa_86c9_d8bf7cd66587  Operator=~=  OutDataTypeStr=boolean  RndMeth=Nearest  InputSameDT=on
  Relational Operator3 : RelationalOperator  RequirementInfo={'other' 'HLSDem_SetPointHi_requirements.docx' '@Simulink_requirement_item_17' 'true' '启用启动状态最高设定转速状态判定' '' } %GIDa_8504bd4b_250f_4fdf_aed0_6c4ae542059a  Operator=<=  OutDataTypeStr=boolean  RndMeth=Nearest  InputSameDT=on
  Switch3 : Switch  Criteria=u2 ~= 0  InputSameDT=on
  HLSDem_stStrt_mp : Outport
  wires:
  Logical Operator4/1 -> HLSDem_stStrt_mp/1  "HLSDem_stStrt_mp"
  CoEng_tiNormal/1 -> Relational Operator3/1
  Relational Operator3/1 -> Logical Operator4/1
  Switch3/1 -> Delay/1, Relational Operator3/2  "HLSDem_tiStrt_mp"
  StSys_stStrt/1 -> Relational Operator1/1
  Constant1/1 -> Relational Operator1/2
  Relational Operator1/1 -> Switch3/2, Logical Operator4/2
  MinMax5/1 -> Switch3/1
  Delay/1 -> Switch3/3
  HLSDem_tiStrtCEngDsT_CUR/1 -> MinMax5/1  "HLSDem_tiStrtCEngDsT_mp"
  HLSDem_tiStrtEngOil_CUR/1 -> MinMax5/2  "HLSDem_tiStrtEngOil_mp"
  CEngDsT_t/1 -> HLSDem_tiStrtCEngDsT_CUR/1
  Oil_tSwmp/1 -> HLSDem_tiStrtEngOil_CUR/1

== system HLSDem_SetPoint/HLSDem_SetPointHi/HLSDem_SetPointBaseHi/Release of reduction ==
  note: %1表示不经过PT1斜坡%
  APP_stKD : Inport
  Gbx_stOvrSpdDem : Inport  Port=2
  Bitwise Operator : simulink/Logic and Bit Operations/Bitwise Operator  logicop=AND  UseBitMask=on  BitMask=bin2dec('00000011')  BitMaskRealWorld=Stored Integer
  Compare To Zero : simulink/Logic and Bit Operations/Compare To Zero  relop=>  OutDataTypeStr=boolean
  Logical Operator3 : Logic  Operator=OR  OutDataTypeStr=boolean
  HLSDem_stNoRmp : Outport
  wires:
  Logical Operator3/1 -> HLSDem_stNoRmp/1  "HLSDem_stNoRmp"
  APP_stKD/1 -> Logical Operator3/1
  Bitwise Operator/1 -> Compare To Zero/1
  Compare To Zero/1 -> Logical Operator3/2
  Gbx_stOvrSpdDem/1 -> Bitwise Operator/1

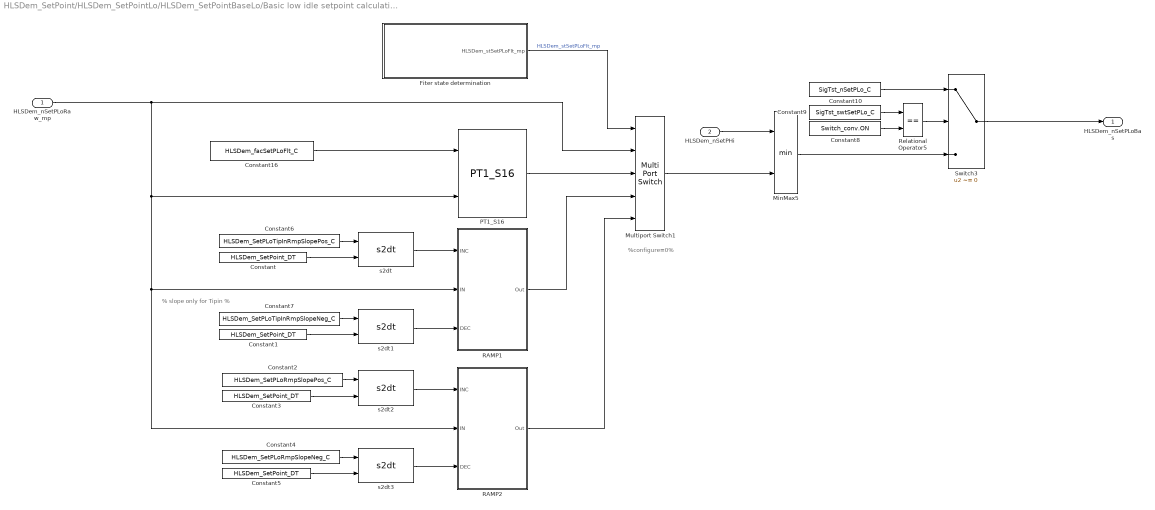
== system HLSDem_SetPoint/HLSDem_SetPointLo/HLSDem_SetPointBaseLo/Basic low idle setpoint calculation ==
  note: % slope only for Tipin %
  note: %configure=0%
  HLSDem_nSetPLoRaw_mp : Inport
  HLSDem_nSetPHi : Inport  Port=2
  Constant{,1,3,5} (4 alike) : Constant  Value=HLSDem_SetPoint_DT
  Constant10 : Constant  RequirementInfo={'other' 'CEngDsT_requirements.doc' '@Simulink_requirement_item_6' 'true' '手动冷却水温值' '' } %GIDa_05ded098_cd89_4260_95da_4b08d6440029  Value=SigTst_nSetPLo_C  SampleTime=-1
  Constant16 : Constant  Value=HLSDem_facSetPLoFlt_C
  Constant2 : Constant  Value=HLSDem_SetPLoRmpSlopePos_C
  Constant4 : Constant  Value=HLSDem_SetPLoRmpSlopeNeg_C
  Constant6 : Constant  Value=HLSDem_SetPLoTipInRmpSlopePos_C
  Constant7 : Constant  Value=HLSDem_SetPLoTipInRmpSlopeNeg_C
  Constant8 : Constant  RequirementInfo={'other' 'APP_requirements.doc' '@Simulink_requirement_item_25' 'true' '手动开关' '' } %GIDa_48448ed4_9fbc_4444_afe2_05043c4178b3  Value=Switch_conv.ON  OutDataTypeStr=Inherit: Inherit via back propagation
  Constant9 : Constant  RequirementInfo={'other' 'CEngDsT_requirements.doc' '@Simulink_requirement_item_6' 'true' '手动冷却水温值' '' } %GIDa_d5f98a65_61c7_4b87_9948_ab5ffe7f2aad  Value=SigTst_swtSetPLo_C  SampleTime=-1
  Fiter state determination : Subsystem
  MinMax5 : MinMax  Inputs=2  SaturateOnIntegerOverflow=on  InputSameDT=on
  Multiport Switch1 : MultiPortSwitch  RequirementInfo={'other' 'HLSDem_SetPointLo_requirements.docx' '@Simulink_requirement_item_20' 'true' '选择目标怠速' '' ; 'other' 'HLSDem_SetPointLo_requirements.docx' '@Simulink_requirement_item_22' 'true' '目标怠速基础值计算' '' } %GIDa_b7737393_141c_43e7_b261_bfac47b1c153  DataPortOrder=Specify indices  Inputs=4  DataPortIndices={3,2,1,0}  DiagnosticForDefault=Warning  SaturateOnIntegerOverflow=on  InputSameDT=on
  PT1_S16 : CXLib/PT1_S16
  RAMP1 : Subsystem
  RAMP2 : Subsystem
  Relational Operator5 : RelationalOperator  Operator===  OutDataTypeStr=boolean  RndMeth=Simplest  InputSameDT=on
  Switch3 : Switch  RequirementInfo={'other' 'CEngDsT_requirements.doc' '@Simulink_requirement_item_6' 'true' '手动冷却水温值' '' } %GIDa_fd964c92_7ec5_495f_8c3c_17833136cee8  Criteria=u2 ~= 0  Threshold=CEngDst_switch_conv.OFF  SaturateOnIntegerOverflow=on  InputSameDT=on
  s2dt{,1..3} (4 alike) : CXLib/s2dt
  HLSDem_nSetPLoBas : Outport
  wires:
  MinMax5/1 -> Switch3/3
  Constant8/1 -> Relational Operator5/2
  Constant9/1 -> Relational Operator5/1
  Relational Operator5/1 -> Switch3/2
  Constant10/1 -> Switch3/1
  Constant5/1 -> s2dt3/2
  Constant3/1 -> s2dt2/2
  Constant4/1 -> s2dt3/1
  Constant2/1 -> s2dt2/1
  s2dt2/1 -> RAMP2/1(INC)
  Constant1/1 -> s2dt1/2
  s2dt/1 -> RAMP1/1(INC)
  Constant/1 -> s2dt/2
  Constant7/1 -> s2dt1/1
  Constant6/1 -> s2dt/1
  Constant16/1 -> PT1_S16/1
  PT1_S16/1 -> Multiport Switch1/3
  RAMP1/1(Out) -> Multiport Switch1/4
  RAMP2/1(Out) -> Multiport Switch1/5
  Fiter state determination/1(HLSDem_stSetPLoFlt_mp) -> Multiport Switch1/1  "HLSDem_stSetPLoFlt_mp"
  Multiport Switch1/1 -> MinMax5/2
  HLSDem_nSetPHi/1 -> MinMax5/1
  Switch3/1 -> HLSDem_nSetPLoBas/1
  HLSDem_nSetPLoRaw_mp/1 -> Multiport Switch1/2, RAMP2/2(IN), RAMP1/2(IN), PT1_S16/2
  s2dt1/1 -> RAMP1/3(DEC)
  s2dt3/1 -> RAMP2/3(DEC)
